simulink model "FRR_3area_6"  (R2015b)
settings: Solver=ode45  StartTime=0.0  StopTime=1000  RelTol=1e-3
values from neighbouring files (symbols this model uses):
  beta = [0.3483 0.3827 0.3692]    [init_FFR_3area.m]    (also in init_FFR_3area_2.m; init_FFR_3area_3.m; init_FFR_3area_4.m; init_FFR_3area_5.m)
  D = 0.015    [init_FFR_1_0.m]    (also in init_FFR_1_1.m; init_FFR_3area.m = [0.015 0.016 0.015]; init_FFR_3area_2.m = [0.015 0.016 0.015]; init_FFR_3area_3.m = [0.015 0.016 0.015])
  H = 0.0833    [init_FFR_1_0.m]    (also in init_FFR_1_1.m; init_FFR_3area.m = [0.1667 0.2017 0.1247] .* 0.5; init_FFR_3area_2.m = [0.1667 0.2017 0.1247] .* 0.5; init_FFR_3area_3.m = [0.1667 0.2017 0.1247] .* 0.5)
  Ki = -0.3    [init_FFR_1_0.m]    (also in init_FFR_1_1.m = -2; init_FFR_3area.m = [-0.3 -0.2 -0.4]; init_FFR_3area_2.m = [-0.3 -0.2 -0.4]; init_FFR_3area_3.m = [-0.3 -0.2 -0.4])
  Kp = -0.5    [init_FFR_1_1.m]    (also in init_FRR_3area_6.m = [-0.5 -0.5 -0.5]; init_FRR_4area_1.m = [0 0 0 0])
  L = 1000    [init_FFR_3area_4.m]    (also in init_FFR_3area_5.m; init_FRR_3area_6.m; init_FRR_4area_1.m)
  MO_down = sortrows(MO_down, 1)    [allocateProduction.m]    (also in init_FFR_3area_4.m; init_FFR_3area_5.m; init_FRR_3area_6.m; init_FRR_4area_1.m)
  MO_up = sortrows(MO_up, 1)    [allocateProduction.m]    (also in init_FFR_3area_4.m; init_FFR_3area_5.m; init_FRR_3area_6.m; init_FRR_4area_1.m)
  R = 3    [init_FFR_1_0.m]    (also in init_FFR_1_1.m; init_FFR_3area.m = [3 2.73 2.82]; init_FFR_3area_2.m = [3 2.73 2.82]; init_FFR_3area_3.m = [3 2.73 2.82])
  sample_time_frr_a = 10    [init_FFR_3area_4.m]    (also in init_FFR_3area_5.m = 2; init_FRR_3area_6.m; init_FRR_4area_1.m)
  T_12 = 0.20    (= 0.2)    [allocateProduction.m]    (also in init_FFR_3area.m; init_FFR_3area_2.m; init_FFR_3area_3.m; init_FFR_3area_4.m)
  T_13 = 0.25    [allocateProduction.m]    (also in init_FFR_3area.m; init_FFR_3area_2.m; init_FFR_3area_3.m; init_FFR_3area_4.m)
  T_21 = 0.20    (= 0.2)    [allocateProduction.m]    (also in init_FFR_3area.m; init_FFR_3area_2.m; init_FFR_3area_3.m; init_FFR_3area_4.m)
  T_23 = 0.12    [allocateProduction.m]    (also in init_FFR_3area.m; init_FFR_3area_2.m; init_FFR_3area_3.m; init_FFR_3area_4.m)
  T_31 = 0.25    [allocateProduction.m]    (also in init_FFR_3area.m; init_FFR_3area_2.m; init_FFR_3area_3.m; init_FFR_3area_4.m)
  T_32 = 0.12    [allocateProduction.m]    (also in init_FFR_3area.m; init_FFR_3area_2.m; init_FFR_3area_3.m; init_FFR_3area_4.m)
  T_g = 0.08    [init_FFR_1_0.m]    (also in init_FFR_1_1.m; init_FFR_3area.m = [0.08 0.06 0.07]; init_FFR_3area_2.m = [0.08 0.06 0.07]; init_FFR_3area_3.m = [0.08 0.06 0.07])
  T_t = 0.40    (= 0.4)    [init_FFR_1_0.m]    (also in init_FFR_1_1.m; init_FFR_3area.m = [0.40 0.44 0.30]; init_FFR_3area_2.m = [0.40 0.44 0.30]; init_FFR_3area_3.m = [0.40 0.44 0.30])
libraries: simulink x6, dspstat3 x1, aerolibanimutils x1
settings Model: Creator=tarje  LastModifiedBy=tarje
settings DataIOCC: SaveFormat=Array
settings HardwareCC: ProdBitPerPointer=32  ProdLargestAtomicFloat=None  ProdIntDivRoundTo=Undefined  ProdEndianess=Unspecified  ProdWordSize=32  ProdHWDeviceType=32-bit Generic
settings GRTTargetCC: GeneratePreprocessorConditionals=Disable all
settings ConfigComp: CovModelRefEnable=Off

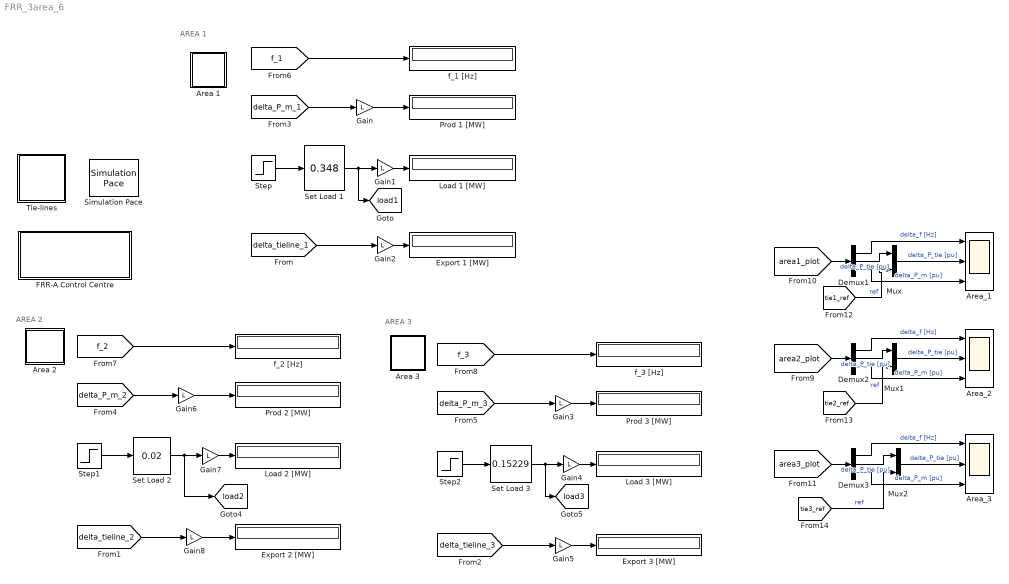
== system FRR_3area_6 ==
  note: AREA 3
  note: AREA 2
  note: AREA 1
  Area 1 : Subsystem
  Area 2 : Subsystem
  Area 3 : Subsystem
  Area_1 : Scope  NumInputPorts=3
  Area_2 : Scope  NumInputPorts=3
  Area_3 : Scope  NumInputPorts=3
  Demux1 : Demux  Outputs=3
  Demux2 : Demux  Outputs=3
  Demux3 : Demux  Outputs=3
  Export 1 [MW] : Display
  Export 2 [MW] : Display
  Export 3 [MW] : Display
  "FRR-A Control Centre " : Subsystem
  Gain{,1..8} (9 alike) : Gain  Gain=L
  Load 1 [MW] : Display
  Load 2 [MW] : Display
  Load 3 [MW] : Display
  Mux : Mux  Inputs=2
  Mux1 : Mux  Inputs=2
  Mux2 : Mux  Inputs=2
  Prod 1 [MW] : Display
  Prod 2 [MW] : Display
  Prod 3 [MW] : Display
  Set Load 1 : simulink/Math Operations/Slider Gain  low=-0.2  gain=0.348  high=0.348
  Set Load 2 : simulink/Math Operations/Slider Gain  low=-0.05  gain=0.02  high=0.348
  Set Load 3 : simulink/Math Operations/Slider Gain  low=-0.05  gain=0.15229  high=1
  Simulation Pace : aerolibanimutils/Simulation Pace  SimulationPace=1  SleepMode=MATLAB Thread  OutputPaceError=off  SampleTime=1/30
      settings: AttributesFormatString=%<SimulationPace> sec/sec
  Step : Step  Time=2  SampleTime=0
  Step1 : Step  Time=2  SampleTime=0
  Step2 : Step  Time=2  SampleTime=0
  Tie-lines : Subsystem
  f_1 [Hz] : Display
  f_2 [Hz] : Display
  f_3 [Hz] : Display
  tag scope: load1=global, load2=global, load3=global
  wires:
  [f_1] -> f_1 [Hz]/1
  [delta_P_m_1] -> Gain/1
  Step/1 -> Set Load 1/1
  Set Load 1/1 -> [load1], Gain1/1
  [f_2] -> f_2 [Hz]/1
  [delta_P_m_2] -> Gain6/1
  Step1/1 -> Set Load 2/1
  Set Load 2/1 -> [load2], Gain7/1
  [f_3] -> f_3 [Hz]/1
  [delta_P_m_3] -> Gain3/1
  Step2/1 -> Set Load 3/1
  Set Load 3/1 -> [load3], Gain4/1
  [delta_tieline_1] -> Gain2/1
  [delta_tieline_2] -> Gain8/1
  [delta_tieline_3] -> Gain5/1
  [area1_plot] -> Demux1/1
  Demux1/1 -> Area_1/1  "delta_f [Hz]"
  Demux1/2 -> Mux/1  "delta_P_tie [pu]"
  Demux1/3 -> Area_1/3  "delta_P_m [pu]"
  [area2_plot] -> Demux2/1
  Demux2/1 -> Area_2/1  "delta_f [Hz]"
  Demux2/2 -> Mux1/1  "delta_P_tie [pu]"
  Demux2/3 -> Area_2/3  "delta_P_m [pu]"
  [area3_plot] -> Demux3/1
  Demux3/1 -> Area_3/1  "delta_f [Hz]"
  Demux3/2 -> Mux2/1  "delta_P_tie [pu]"
  Demux3/3 -> Area_3/3  "delta_P_m [pu]"
  Mux/1 -> Area_1/2  "delta_P_tie [pu]"
  [tie1_ref] -> Mux/2  "ref"
  [tie2_ref] -> Mux1/2  "ref"
  Mux1/1 -> Area_2/2  "delta_P_tie [pu]"
  Mux2/1 -> Area_3/2  "delta_P_tie [pu]"
  [tie3_ref] -> Mux2/2  "ref"
  Gain/1 -> Prod 1 [MW]/1
  Gain1/1 -> Load 1 [MW]/1
  Gain2/1 -> Export 1 [MW]/1
  Gain3/1 -> Prod 3 [MW]/1
  Gain4/1 -> Load 3 [MW]/1
  Gain5/1 -> Export 3 [MW]/1
  Gain6/1 -> Prod 2 [MW]/1
  Gain7/1 -> Load 2 [MW]/1
  Gain8/1 -> Export 2 [MW]/1

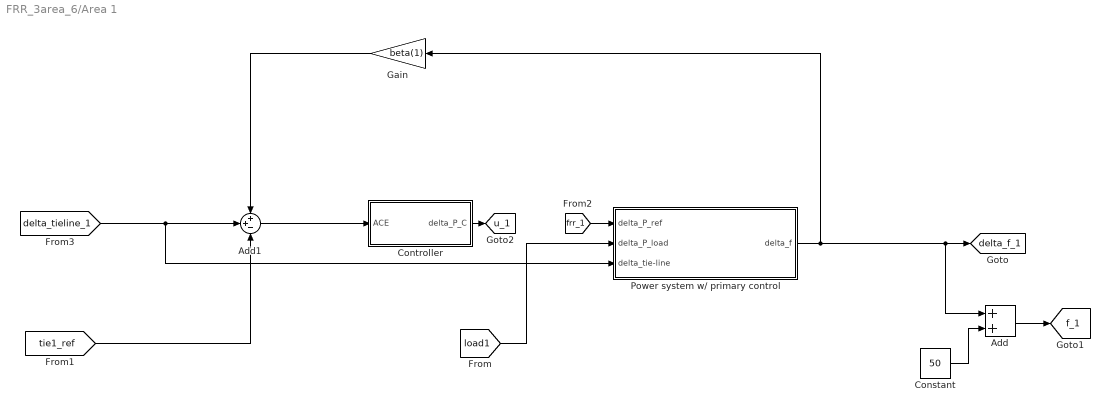
== system FRR_3area_6/Area 1 ==
  Add : Sum
  Add1 : Sum  Inputs=++-
  Constant : Constant  Value=50
  Controller : Subsystem  SystemSampleTime=sample_time_frr_a
  Gain : Gain  Gain=beta(1)
  Power system w/ primary control : Subsystem
  tag scope: delta_f_1=global, f_1=global, u_1=global
  wires:
  Power system w/ primary control/1(delta_f) -> [delta_f_1], Add/1, Gain/1
  Constant/1 -> Add/2
  Add/1 -> [f_1]
  [tie1_ref] -> Add1/3
  Add1/1 -> Controller/1(ACE)
  [load1] -> Power system w/ primary control/2(delta_P_load)
  [delta_tieline_1] -> Power system w/ primary control/3(delta_tie-line), Add1/2
  Gain/1 -> Add1/1
  [frr_1] -> Power system w/ primary control/1(delta_P_ref)
  Controller/1(delta_P_C) -> [u_1]

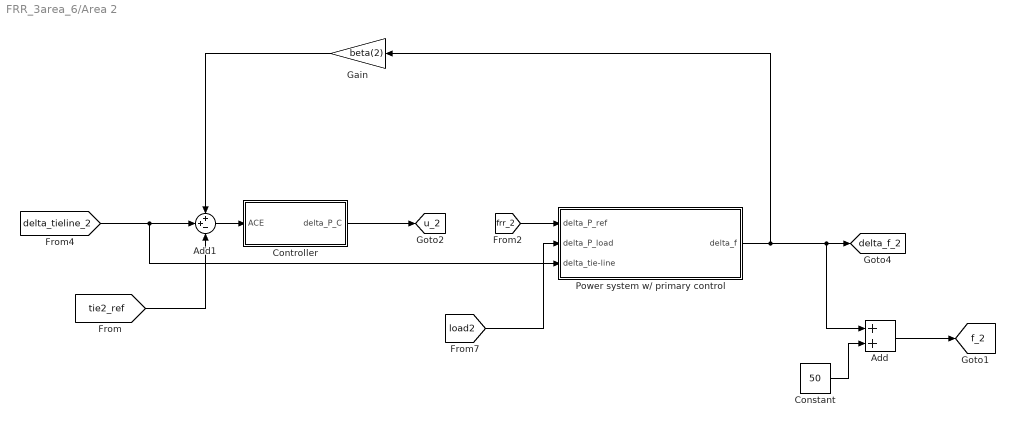
== system FRR_3area_6/Area 2 ==
  Add : Sum
  Add1 : Sum  Inputs=++-
  Constant : Constant  Value=50
  Controller : Subsystem  SystemSampleTime=sample_time_frr_a
  Gain : Gain  Gain=beta(2)
  Power system w/ primary control : Subsystem
  tag scope: delta_f_2=global, f_2=global, u_2=global
  wires:
  Power system w/ primary control/1(delta_f) -> Add/1, [delta_f_2], Gain/1
  Constant/1 -> Add/2
  Add/1 -> [f_2]
  [tie2_ref] -> Add1/3
  [load2] -> Power system w/ primary control/2(delta_P_load)
  Add1/1 -> Controller/1(ACE)
  [delta_tieline_2] -> Power system w/ primary control/3(delta_tie-line), Add1/2
  Gain/1 -> Add1/1
  Controller/1(delta_P_C) -> [u_2]
  [frr_2] -> Power system w/ primary control/1(delta_P_ref)

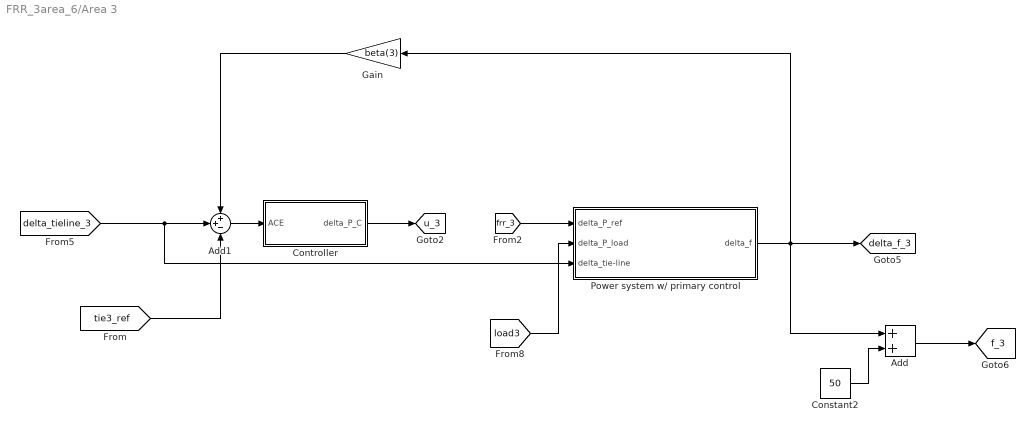
== system FRR_3area_6/Area 3 ==
  Add : Sum
  Add1 : Sum  Inputs=++-
  Constant2 : Constant  Value=50
  Controller : Subsystem  SystemSampleTime=sample_time_frr_a
  Gain : Gain  Gain=beta(3)
  Power system w/ primary control : Subsystem
  tag scope: delta_f_3=global, f_3=global, u_3=global
  wires:
  Power system w/ primary control/1(delta_f) -> [delta_f_3], Add/1, Gain/1
  Add/1 -> [f_3]
  Constant2/1 -> Add/2
  [tie3_ref] -> Add1/3
  [load3] -> Power system w/ primary control/2(delta_P_load)
  Add1/1 -> Controller/1(ACE)
  [delta_tieline_3] -> Power system w/ primary control/3(delta_tie-line), Add1/2
  Gain/1 -> Add1/1
  Controller/1(delta_P_C) -> [u_3]
  [frr_3] -> Power system w/ primary control/1(delta_P_ref)

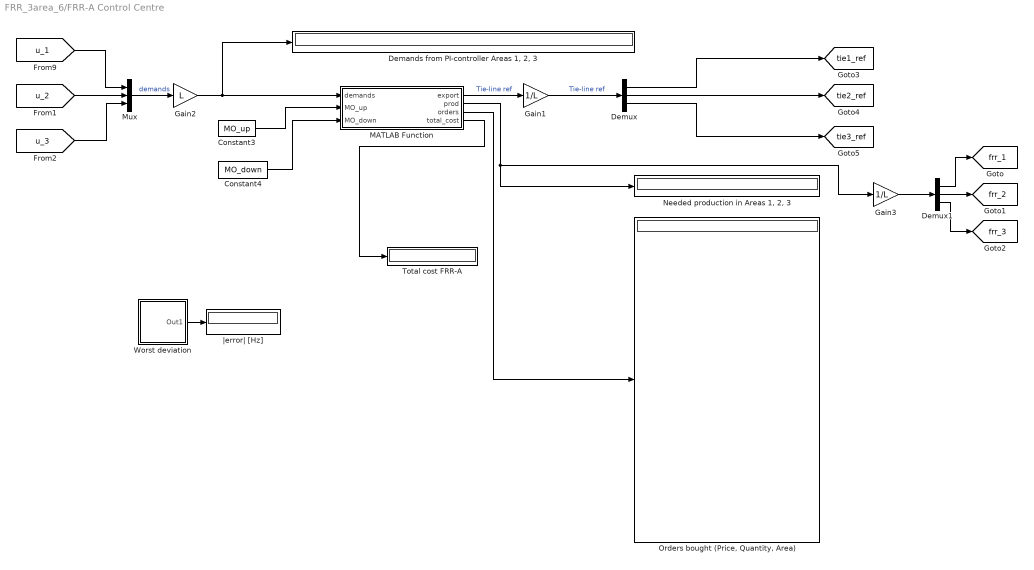
== system FRR_3area_6/FRR-A Control Centre  ==
  Constant3 : Constant  Value=MO_up
  Constant4 : Constant  Value=MO_down
  "Demands from PI-controller Areas 1, 2, 3" : Display
  Demux : Demux  Outputs=3
  Demux1 : Demux  Outputs=3
  Gain1 : Gain  Gain=1/L
  Gain2 : Gain  Gain=L
  Gain3 : Gain  Gain=1/L
  MATLAB Function : MATLAB Function  TreatAsAtomicUnit=on  SystemSampleTime=sample_time_frr_a
  Mux : Mux  Inputs=3
  "Needed production in Areas 1, 2, 3" : Display
  "Orders bought (Price, Quantity, Area)" : Display
  Total cost FRR-A : Display
      settings: Format=bank
  Worst deviation : Subsystem
  |error| [Hz] : Display
  tag scope: frr_1=global, frr_2=global, frr_3=global, tie1_ref=global, tie2_ref=global, tie3_ref=global
  wires:
  Gain1/1 -> Demux/1  "Tie-line ref"
  Constant3/1 -> MATLAB Function/2(MO_up)
  Constant4/1 -> MATLAB Function/3(MO_down)
  Demux/1 -> [tie1_ref]
  Demux/2 -> [tie2_ref]
  Demux/3 -> [tie3_ref]
  MATLAB Function/3(orders) -> "Orders bought (Price, Quantity, Area)"/1
  MATLAB Function/4(total_cost) -> Total cost FRR-A/1
  Gain2/1 -> "Demands from PI-controller Areas 1, 2, 3"/1, MATLAB Function/1(demands)
  Mux/1 -> Gain2/1  "demands"
  [u_1] -> Mux/1
  [u_2] -> Mux/2
  [u_3] -> Mux/3
  MATLAB Function/2(prod) -> Gain3/1, "Needed production in Areas 1, 2, 3"/1
  Demux1/1 -> [frr_1]
  Demux1/2 -> [frr_2]
  Demux1/3 -> [frr_3]
  Gain3/1 -> Demux1/1
  Worst deviation/1(Out1) -> |error| [Hz]/1
  MATLAB Function/1(export) -> Gain1/1  "Tie-line ref"

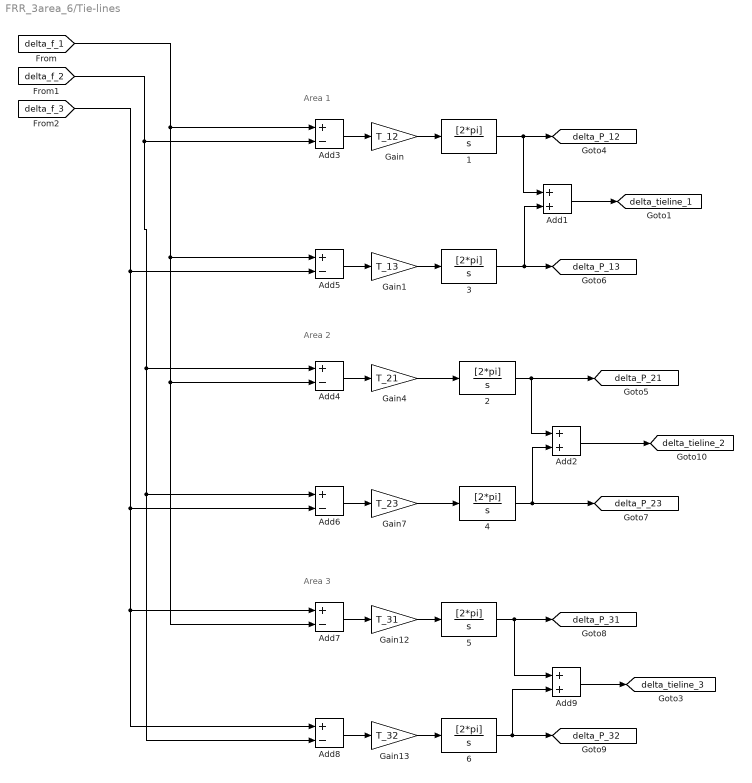
== system FRR_3area_6/Tie-lines ==
  note: Area 3
  note: Area 2
  note: Area 1
   {1..6} (6 alike) : TransferFcn  Numerator=[2*pi]  Denominator=[1 0]
  Add1 : Sum
  Add2 : Sum
  Add{3..8} (6 alike) : Sum  Inputs=+-
  Add9 : Sum
  Gain : Gain  Gain=T_12
  Gain1 : Gain  Gain=T_13
  Gain12 : Gain  Gain=T_31
  Gain13 : Gain  Gain=T_32
  Gain4 : Gain  Gain=T_21
  Gain7 : Gain  Gain=T_23
  tag scope: delta_P_12=global, delta_P_13=global, delta_P_21=global, delta_P_23=global, delta_P_31=global, delta_P_32=global, delta_tieline_1=global, delta_tieline_2=global, delta_tieline_3=global
  wires:
  [delta_f_2] -> Add3/2, Add8/2, Add6/1, Add4/1
  [delta_f_1] -> Add3/1, Add5/1, Add7/2, Add4/2
  [delta_f_3] -> Add5/2, Add8/1, Add7/1, Add6/2
  " 1"/1 -> Add1/1, [delta_P_12]
  Add3/1 -> Gain/1
  " 2"/1 -> Add2/1, [delta_P_21]
  Add4/1 -> Gain4/1
  " 3"/1 -> Add1/2, [delta_P_13]
  Add5/1 -> Gain1/1
  " 4"/1 -> Add2/2, [delta_P_23]
  Add6/1 -> Gain7/1
  " 5"/1 -> Add9/1, [delta_P_31]
  Add7/1 -> Gain12/1
  " 6"/1 -> Add9/2, [delta_P_32]
  Add8/1 -> Gain13/1
  Add9/1 -> [delta_tieline_3]
  Gain12/1 -> " 5"/1
  Gain13/1 -> " 6"/1
  Add2/1 -> [delta_tieline_2]
  Gain4/1 -> " 2"/1
  Gain7/1 -> " 4"/1
  Add1/1 -> [delta_tieline_1]
  Gain/1 -> " 1"/1
  Gain1/1 -> " 3"/1

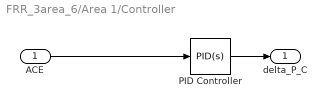
== system FRR_3area_6/Area 1/Controller ==
  ACE : Inport
  PID Controller : simulink/Continuous/PID Controller  Controller=PID  TimeDomain=Continuous-time  SampleTime=-1  IntegratorMethod=Forward Euler  FilterMethod=Forward Euler  Form=Parallel  UseFilter=on  ControllerParametersSource=internal  P=Kp(1)  I=Ki(1)  D=0  N=0  InitialConditionSource=internal  InitialConditionForIntegrator=0  InitialConditionForFilter=0  ExternalReset=none  LimitOutput=off  UpperSaturationLimit=inf  LowerSaturationLimit=-inf  LinearizeAsGain=on  AntiWindupMode=none  Kb=1  TrackingMode=off  Kt=1  PParamMin=[]  PParamMax=[]  IParamMin=[]  IParamMax=[]  DParamMin=[]  DParamMax=[]  NParamMin=[]  NParamMax=[]  KbParamMin=[]  KbParamMax=[]  KtParamMin=[]  KtParamMax=[]  POutMin=[]  POutMax=[]  IOutMin=[]  IOutMax=[]  DOutMin=[]  DOutMax=[]  NOutMin=[]  NOutMax=[]  KbOutMin=[]  KbOutMax=[]  KtOutMin=[]  KtOutMax=[]  IntegratorOutMin=[]  IntegratorOutMax=[]  FilterOutMin=[]  FilterOutMax=[]  SumOutMin=[]  SumOutMax=[]  SumI1OutMin=[]  SumI1OutMax=[]  SumI2OutMin=[]  SumI2OutMax=[]  SumI3OutMin=[]  SumI3OutMax=[]  SumDOutMin=[]  SumDOutMax=[]  SaturationOutMin=[]  SaturationOutMax=[]  IntegratorContinuousStateAttributes=''  IntegratorStateMustResolveToSignalObject=off  IntegratorRTWStateStorageClass=Auto  FilterContinuousStateAttributes=''  FilterStateMustResolveToSignalObject=off  FilterRTWStateStorageClass=Auto  DifferentiatorICPrevScaledInput=0  DifferentiatorOutMin=[]  DifferentiatorOutMax=[]
  delta_P_C : Outport
  wires:
  PID Controller/1 -> delta_P_C/1
  ACE/1 -> PID Controller/1

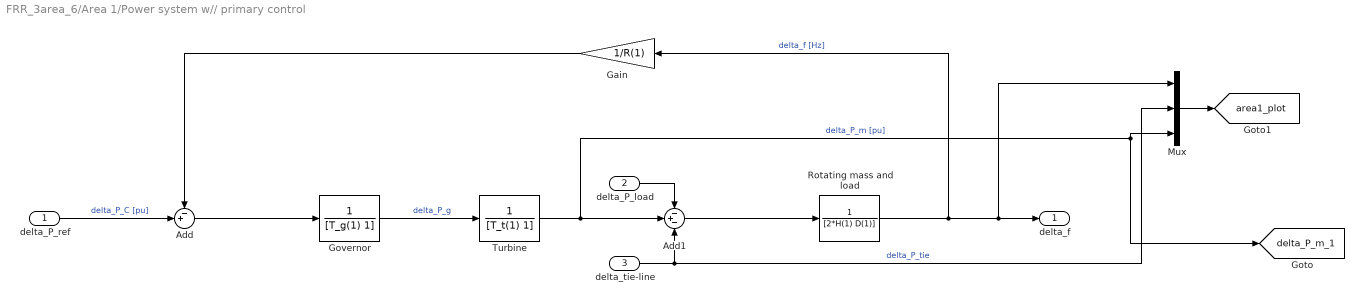
== system FRR_3area_6/Area 1/Power system w// primary control ==
  delta_P_ref : Inport
  delta_P_load : Inport  Port=2
  delta_tie-line : Inport  Port=3
  Add : Sum  Inputs=-+|
  Add1 : Sum  Inputs=-+-
  Gain : Gain  Gain=1/R(1)
  Governor : TransferFcn  Denominator=[T_g(1) 1]
  Mux : Mux  Inputs=3
  Rotating mass and load : TransferFcn  Denominator=[2*H(1) D(1)]
  Turbine : TransferFcn  Denominator=[T_t(1) 1]
  delta_f : Outport
  tag scope: area1_plot=global, delta_P_m_1=global
  wires:
  Turbine/1 -> Mux/3, [delta_P_m_1], Add1/2  "delta_P_m [pu]"
  Rotating mass and load/1 -> Mux/1, delta_f/1, Gain/1  "delta_f [Hz]"
  Gain/1 -> Add/1
  Add1/1 -> Rotating mass and load/1
  Add/1 -> Governor/1
  Governor/1 -> Turbine/1  "delta_P_g"
  delta_P_ref/1 -> Add/2  "delta_P_C [pu]"
  delta_P_load/1 -> Add1/1
  delta_tie-line/1 -> Mux/2, Add1/3  "delta_P_tie"
  Mux/1 -> [area1_plot]

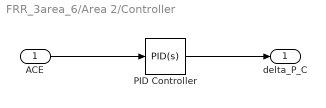
== system FRR_3area_6/Area 2/Controller ==
  ACE : Inport
  PID Controller : simulink/Continuous/PID Controller  Controller=PID  TimeDomain=Continuous-time  SampleTime=-1  IntegratorMethod=Forward Euler  FilterMethod=Forward Euler  Form=Parallel  UseFilter=on  ControllerParametersSource=internal  P=Kp(2)  I=Ki(2)  D=0  N=100  InitialConditionSource=internal  InitialConditionForIntegrator=0  InitialConditionForFilter=0  ExternalReset=none  LimitOutput=off  UpperSaturationLimit=inf  LowerSaturationLimit=-inf  LinearizeAsGain=on  AntiWindupMode=none  Kb=1  TrackingMode=off  Kt=1  PParamMin=[]  PParamMax=[]  IParamMin=[]  IParamMax=[]  DParamMin=[]  DParamMax=[]  NParamMin=[]  NParamMax=[]  KbParamMin=[]  KbParamMax=[]  KtParamMin=[]  KtParamMax=[]  POutMin=[]  POutMax=[]  IOutMin=[]  IOutMax=[]  DOutMin=[]  DOutMax=[]  NOutMin=[]  NOutMax=[]  KbOutMin=[]  KbOutMax=[]  KtOutMin=[]  KtOutMax=[]  IntegratorOutMin=[]  IntegratorOutMax=[]  FilterOutMin=[]  FilterOutMax=[]  SumOutMin=[]  SumOutMax=[]  SumI1OutMin=[]  SumI1OutMax=[]  SumI2OutMin=[]  SumI2OutMax=[]  SumI3OutMin=[]  SumI3OutMax=[]  SumDOutMin=[]  SumDOutMax=[]  SaturationOutMin=[]  SaturationOutMax=[]  IntegratorContinuousStateAttributes=''  IntegratorStateMustResolveToSignalObject=off  IntegratorRTWStateStorageClass=Auto  FilterContinuousStateAttributes=''  FilterStateMustResolveToSignalObject=off  FilterRTWStateStorageClass=Auto  DifferentiatorICPrevScaledInput=0  DifferentiatorOutMin=[]  DifferentiatorOutMax=[]
  delta_P_C : Outport
  wires:
  PID Controller/1 -> delta_P_C/1
  ACE/1 -> PID Controller/1

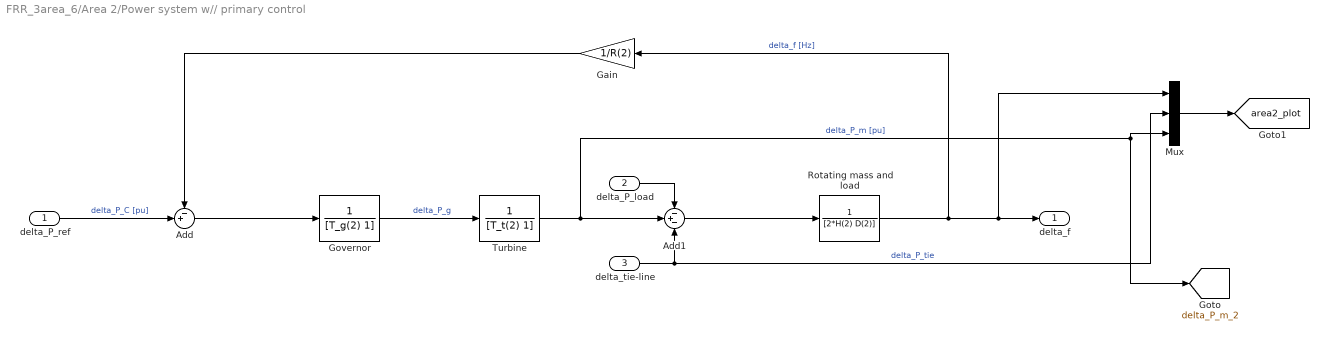
== system FRR_3area_6/Area 2/Power system w// primary control ==
  delta_P_ref : Inport
  delta_P_load : Inport  Port=2
  delta_tie-line : Inport  Port=3
  Add : Sum  Inputs=-+|
  Add1 : Sum  Inputs=-+-
  Gain : Gain  Gain=1/R(2)
  Governor : TransferFcn  Denominator=[T_g(2) 1]
  Mux : Mux  Inputs=3
  Rotating mass and load : TransferFcn  Denominator=[2*H(2) D(2)]
  Turbine : TransferFcn  Denominator=[T_t(2) 1]
  delta_f : Outport
  tag scope: area2_plot=global, delta_P_m_2=global
  wires:
  Turbine/1 -> Mux/3, [delta_P_m_2], Add1/2  "delta_P_m [pu]"
  Rotating mass and load/1 -> Mux/1, delta_f/1, Gain/1  "delta_f [Hz]"
  Gain/1 -> Add/1
  Add1/1 -> Rotating mass and load/1
  Add/1 -> Governor/1
  Governor/1 -> Turbine/1  "delta_P_g"
  delta_P_ref/1 -> Add/2  "delta_P_C [pu]"
  delta_P_load/1 -> Add1/1
  delta_tie-line/1 -> Mux/2, Add1/3  "delta_P_tie"
  Mux/1 -> [area2_plot]

== system FRR_3area_6/Area 3/Controller ==
  ACE : Inport
  PID Controller : simulink/Continuous/PID Controller  Controller=PID  TimeDomain=Continuous-time  SampleTime=-1  IntegratorMethod=Forward Euler  FilterMethod=Forward Euler  Form=Parallel  UseFilter=on  ControllerParametersSource=internal  P=Kp(3)  I=Ki(3)  D=0  N=100  InitialConditionSource=internal  InitialConditionForIntegrator=0  InitialConditionForFilter=0  ExternalReset=none  LimitOutput=off  UpperSaturationLimit=inf  LowerSaturationLimit=-inf  LinearizeAsGain=on  AntiWindupMode=none  Kb=1  TrackingMode=off  Kt=1  PParamMin=[]  PParamMax=[]  IParamMin=[]  IParamMax=[]  DParamMin=[]  DParamMax=[]  NParamMin=[]  NParamMax=[]  KbParamMin=[]  KbParamMax=[]  KtParamMin=[]  KtParamMax=[]  POutMin=[]  POutMax=[]  IOutMin=[]  IOutMax=[]  DOutMin=[]  DOutMax=[]  NOutMin=[]  NOutMax=[]  KbOutMin=[]  KbOutMax=[]  KtOutMin=[]  KtOutMax=[]  IntegratorOutMin=[]  IntegratorOutMax=[]  FilterOutMin=[]  FilterOutMax=[]  SumOutMin=[]  SumOutMax=[]  SumI1OutMin=[]  SumI1OutMax=[]  SumI2OutMin=[]  SumI2OutMax=[]  SumI3OutMin=[]  SumI3OutMax=[]  SumDOutMin=[]  SumDOutMax=[]  SaturationOutMin=[]  SaturationOutMax=[]  IntegratorContinuousStateAttributes=''  IntegratorStateMustResolveToSignalObject=off  IntegratorRTWStateStorageClass=Auto  FilterContinuousStateAttributes=''  FilterStateMustResolveToSignalObject=off  FilterRTWStateStorageClass=Auto  DifferentiatorICPrevScaledInput=0  DifferentiatorOutMin=[]  DifferentiatorOutMax=[]
  delta_P_C : Outport
  wires:
  PID Controller/1 -> delta_P_C/1
  ACE/1 -> PID Controller/1

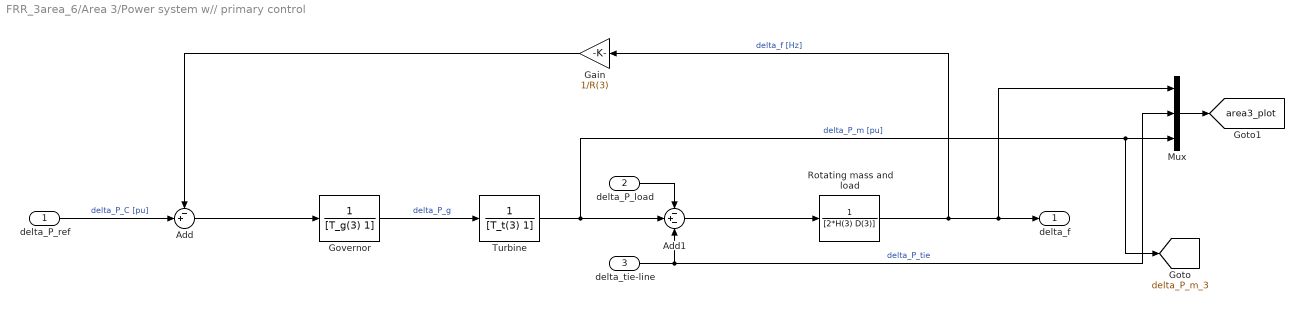
== system FRR_3area_6/Area 3/Power system w// primary control ==
  delta_P_ref : Inport
  delta_P_load : Inport  Port=2
  delta_tie-line : Inport  Port=3
  Add : Sum  Inputs=-+|
  Add1 : Sum  Inputs=-+-
  Gain : Gain  Gain=1/R(3)
  Governor : TransferFcn  Denominator=[T_g(3) 1]
  Mux : Mux  Inputs=3
  Rotating mass and load : TransferFcn  Denominator=[2*H(3) D(3)]
  Turbine : TransferFcn  Denominator=[T_t(3) 1]
  delta_f : Outport
  tag scope: area3_plot=global, delta_P_m_3=global
  wires:
  Turbine/1 -> [delta_P_m_3], Mux/3, Add1/2  "delta_P_m [pu]"
  Rotating mass and load/1 -> Mux/1, delta_f/1, Gain/1  "delta_f [Hz]"
  Gain/1 -> Add/1
  Add1/1 -> Rotating mass and load/1
  Add/1 -> Governor/1
  Governor/1 -> Turbine/1  "delta_P_g"
  delta_P_ref/1 -> Add/2  "delta_P_C [pu]"
  delta_P_load/1 -> Add1/1
  delta_tie-line/1 -> Mux/2, Add1/3  "delta_P_tie"
  Mux/1 -> [area3_plot]

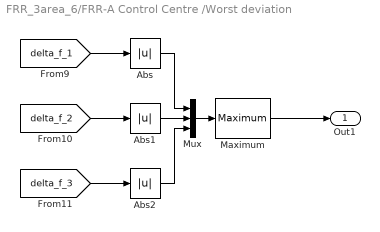
== system FRR_3area_6/FRR-A Control Centre /Worst deviation ==
  Abs : Abs
  Abs1 : Abs
  Abs2 : Abs
  Maximum : dspstat3/Maximum  fcn=Value  reset=None  InputProcessing=Columns as channels (frame based)  indexBase=One  operateOver=Each column  Dimension=1  operation=maximum  roiEnable=off  roiType=Rectangles  roiPortion=Entire ROI  roiOutput=Individual statistics for each ROI  roiFlag=off  accumDataTypeStr=Inherit: Same as product output  accumLastDataTypeStr=Inherit: Same as product output  roundingMode=Ceiling  overflowMode=off
  Mux : Mux  Inputs=3
  Out1 : Outport
  wires:
  Maximum/1 -> Out1/1
  Abs2/1 -> Mux/3
  Mux/1 -> Maximum/1
  [delta_f_2] -> Abs1/1
  [delta_f_3] -> Abs2/1
  Abs/1 -> Mux/1
  Abs1/1 -> Mux/2
  [delta_f_1] -> Abs/1

== matlab function FRR_3area_6/FRR-A Control Centre /MATLAB Function ==
  data: demands input; export output size=3; prod output; MO_up input; MO_down input; orders output; total_cost output
function [export, prod, orders, total_cost] = meritOrder(demands, MO_up, MO_down)

% Define variables
PRICE = 1;
QUANTITY = 2;
AREA = 3;
LEFT = 4;

prod = zeros(length(demands),1);

% Sum demands
demand = sum(demands);
orders = zeros(max(length(MO_up),length(MO_down)),3);

% If frequency is too low
if demand >= 0
    % Check if MO_up is empty
    % orders = zeros(length(MO_up),3); % Declare max size of orders output
    for i = 1:length(MO_up)
        q = MO_up(i, QUANTITY);
        if demand > q
            prod(MO_up(i,AREA)) = prod(MO_up(i,AREA)) + q;
            orders(i,:) = MO_up(i,:);
            demand = demand - q;
        else
            prod(MO_up(i,AREA)) = prod(MO_up(i,AREA)) + demand;
            orders(i,:) = MO_up(i,:);
            orders(i,QUANTITY) = demand;
            demand = 0;
            break;
        end
    end
    if demand ~= 0
        % Not enough UP-bids
    end
% If frequency is too high
else
    demand = abs(demand); % Change sign of demand
    % Check if MO_down is empty
    for i = 1:length(MO_down)
        q = MO_down(i, QUANTITY);
        if demand > q
            prod(MO_down(i,AREA)) = prod(MO_down(i,AREA)) - q;
            orders(i,:) = MO_down(i,:);
            demand = demand - q;
        else
            prod(MO_down(i,AREA)) = prod(MO_down(i,AREA)) - demand;
            orders(i,:) = MO_down(i,:);
            orders(i,QUANTITY) = demand;
            demand = 0;
            break;
        end
    end
    if demand ~= 0
        % Not enough DOWN-bids
    end
end

% Find flow between areas
export = prod - demands;


% Find total cost
total_cost = 0;
for i = 1:length(orders)
    total_cost = total_cost + orders(i,PRICE) * orders(i,QUANTITY);
end
